simulink model "DPLL_1st_Order"  (R2019b)
settings: Solver=VariableStepAuto  StartTime=0.0  StopTime=0.001  MaxStep=1e-6  RelTol=1e-3
libraries: dspfdesign x1, dspsigops x1, dspsrcs4 x1
settings Model: Creator=taiya  LastModifiedBy=taiya

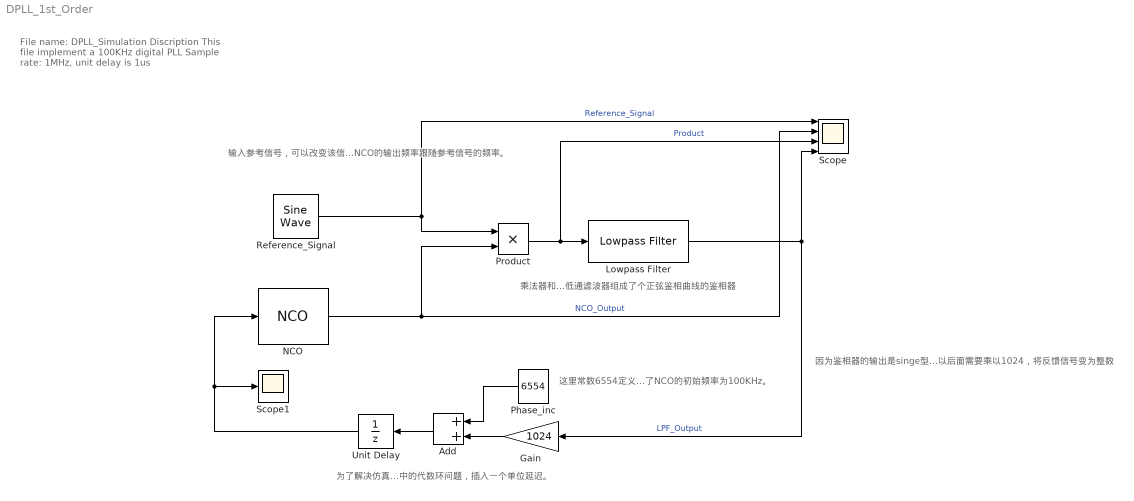
== system DPLL_1st_Order ==
  note: 因为鉴相器的输出是singe型的，值域为[-1,1]，所以后面需要乘以1024，将反馈信号变为整数
  note: 为了解决仿真中的代数环问题，插入一个单位延迟。
  note: 输入参考信号，可以改变该信号的频率，使NCO的输出频率跟随参考信号的频率。
  note: 乘法器和低通滤波器组成了个正弦鉴相曲线的鉴相器
  note: 这里常数6554定义了NCO的初始频率为100KHz。
  note: File name: DPLL_Simulation
      | Discription
      | This file implement a 100KHz digital PLL
      | Sample rate: 1MHz, unit delay is 1us
  Add : Sum
  Gain : Gain  Gain=1024  OutDataTypeStr=int16
  Lowpass Filter : dspfdesign/Lowpass Filter  FilterType=FIR  DesignForMinimumOrder=on  FilterOrder=50  PassbandFrequency=10e3  StopbandFrequency=50e3  PassbandRipple=0.1  StopbandAttenuation=30  InheritSampleRate=off  SampleRate=1e6  SimulateUsing=Interpreted execution  roundingMode=Floor  coeffsDataTypeStr=fixdt(1,16)
  NCO : dspsigops/NCO  AccIncSrc=Input port  AccInc=100  PhaseOffsetSrc=Specify via dialog  PhaseOffset=0  AccumWL=16  HasDither=on  DitherWL=4  PNgeneratorLength=19  HasPhaseQuantizer=on  TableDepth=12  HasOutputPhaseError=off  Formula=Sine  DataType=single  OutputWL=16  OutputFL=14  CompMethod=Table lookup (no interpolation)  SampleTime=1  SamplesPerFrame=1  OutputFrames=off
      settings: SourceProductName=DSP System Toolbox  SourceProductBaseCode=DS
  Phase_inc : Constant  Value=6554  VectorParams1D=off  OutDataTypeStr=int16  SampleTime=1e-6
  Product : Product
  Reference_Signal : dspsrcs4/Sine Wave  Amplitude=1  Frequency=99e3  Phase=0  SampleMode=Discrete  OutComplex=Real  CompMethod=Trigonometric fcn  TableSize=Speed  SampleTime=1e-6  SamplesPerFrame=1  ResetState=Restart at time zero  OutputFrames=off  dataType=single  wordLen=16  udDataType=sfix(16)  fracBitsMode=Best precision  numFracBits=15  OutDataTypeStr=single  LastOutDataTypeStr=single
  Scope : Scope  NumInputPorts=4
  Scope1 : Scope
  Unit Delay : UnitDelay  SampleTime=-1  HasFrameUpgradeWarning=on
  wires:
  NCO/1 -> Product/2, Scope/2  "NCO_Output"
  Reference_Signal/1 -> Product/1, Scope/1  "Reference_Signal"
  Product/1 -> Lowpass Filter/1, Scope/3  "Product"
  Lowpass Filter/1 -> Gain/1, Scope/4  "LPF_Output"
  Gain/1 -> Add/2
  Phase_inc/1 -> Add/1
  Add/1 -> Unit Delay/1
  Unit Delay/1 -> Scope1/1, NCO/1
